simulink model "mpc_output_constr"  (Simulink 6.0)
settings: Solver=ode45  SolverMode=SingleTasking  StartTime=0.0  StopTime=Tstop  RelTol=1e-3
values from neighbouring files (symbols this model uses):
  A = [-.0151 -60.5651 0 -32.174 ... (first row only)    [afti16.m]    (also in misoss.m = sys.a)
  B = [-2.516 -13.136 ... (first row only)    [afti16.m]    (also in misoss.m = sys.b)
  C = [0 1 0 0 ... (first row only)    [afti16.m]    (also in misoss.m = sys.c)
  D = [0 0 ... (first row only)    [afti16.m]    (also in misoss.m = sys.d)
  x0 = zeros(4,1)    [afti16.m]    (also in misoss.m = [0 0 0 0 0]'; mpcrtwdemo.m = [0 0]')
libraries: mpclib x1
settings Model: Creator=jowen  LastModifiedBy=jowen  ExtModeTrigMode=oneshot  ExtModeArmWhenConnect=off
settings DataIOCC: LimitDataPoints=off  SignalLoggingName=sigsOut
settings OptimizationCC: BooleanDataType=off
settings DebuggingCC: CheckExecutionContextPreStartOutputMsg=on  CheckExecutionContextRuntimeOutputMsg=on  SolverPrmCheckMsg=none  IntegerOverflowMsg=none
settings HardwareCC: TargetUnknown=on
settings SFSimCC: SFSimApplyToAllLibs=on  SFSimBuildMode=Incremental

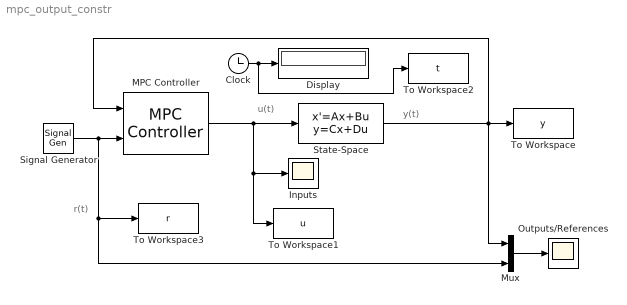
== system mpc_output_constr ==
  note: u(t)
  note: y(t)
  note: r(t)
  Clock : Clock
      settings: Decimation=10
  Display : Display
  Inputs : Scope
      settings: TimeRange=10  YMin=-1.5  YMax=1.5  DataFormat=Structure
  MPC Controller : mpclib/MPC Controller  mpcobj=mpccon  n_mv=0  x0=[]  ref_from_ws=off  ref_signal_name=[]  ref_preview=on  md_from_ws=off  md_signal_name=[]  md_preview=on  from_project=off  md_inport=off  project_file=MPCtask.mat
  Mux : Mux  Inputs=2
  Outputs/References : Scope
      settings: TimeRange=10  YMin=-1  YMax=1  DataFormat=Structure
  Signal Generator : SignalGenerator  Frequency=.4
  State-Space : StateSpace  A=A  B=B  C=C  D=D  X0=x0
  To Workspace : ToWorkspace  VariableName=y  SampleTime=-1  SaveFormat=Array
      settings: MaxDataPoints=Inf
  To Workspace1 : ToWorkspace  VariableName=u  SampleTime=-1  SaveFormat=Array
      settings: MaxDataPoints=Inf
  To Workspace2 : ToWorkspace  VariableName=t  SampleTime=-1  SaveFormat=Array
      settings: MaxDataPoints=Inf
  To Workspace3 : ToWorkspace  VariableName=r  SampleTime=-1  SaveFormat=Array
      settings: MaxDataPoints=Inf
  wires:
  MPC Controller/1 -> State-Space/1, Inputs/1, To Workspace1/1
  State-Space/1 -> To Workspace/1, Mux/1, MPC Controller/1
  Mux/1 -> Outputs/References/1
  Signal Generator/1 -> Mux/2, To Workspace3/1, MPC Controller/2
  Clock/1 -> Display/1, To Workspace2/1
